simulink model "backlashcomptest"  (R2016a)
settings: Solver=VariableStepAuto  StartTime=0.0  StopTime=100  RelTol=1e-3
settings Model: Creator=julianleland  LastModifiedBy=julianleland

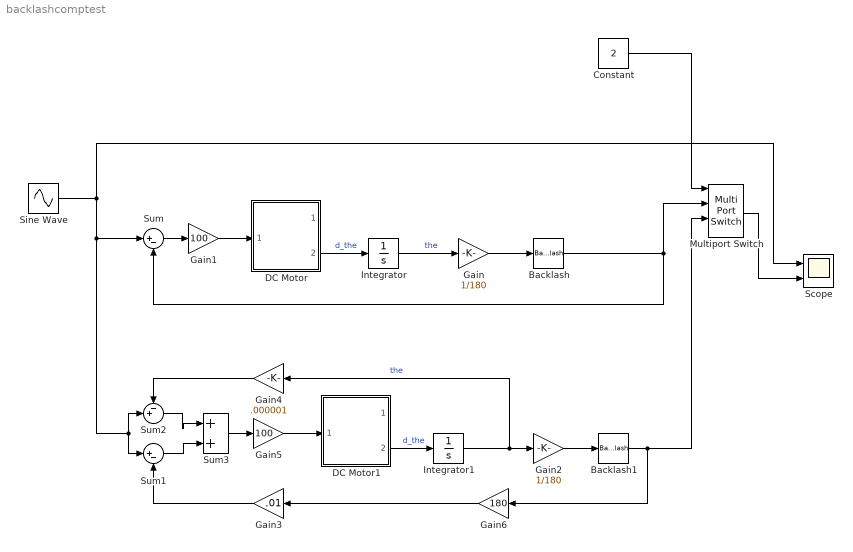
== system backlashcomptest ==
  Backlash : Backlash  BacklashWidth=10
  Backlash1 : Backlash  BacklashWidth=10
  Constant : Constant  Value=2
  DC Motor : Subsystem  mask(DC Motor){R=1, L=1, Q=2}
      mask prompts: R "Winding Resistance (ohms)"; L "Winding Inductance (mH)"; Q "Q Variable"
      mask help: From MIT Simulink Tutorial IAP 2017, Session 2. Provides basic model of DC motor using Kirchoff & Newton's laws.
      mask init:
      | J = R*L/Q
      | b = 1
      | k = 1
      | K = 1
      mask Help: See Julian with questions.
  DC Motor1 : Subsystem  mask(DC Motor){R=1, L=1, Q=2}
      mask prompts: R "Winding Resistance (ohms)"; L "Winding Inductance (mH)"; Q "Q Variable"
      mask help: From MIT Simulink Tutorial IAP 2017, Session 2. Provides basic model of DC motor using Kirchoff & Newton's laws.
      mask init:
      | J = R*L/Q
      | b = 1
      | k = 1
      | K = 1
      mask Help: See Julian with questions.
  Gain : Gain  Gain=1/180
  Gain1 : Gain  Gain=100
  Gain2 : Gain  Gain=1/180
  Gain3 : Gain  Gain=.01
  Gain4 : Gain  Gain=.000001
  Gain5 : Gain  Gain=100
  Gain6 : Gain  Gain=180
  Integrator : Integrator
  Integrator1 : Integrator
  Multiport Switch : MultiPortSwitch
  Scope : Scope  NumInputPorts=2
  Sine Wave : Sin  Amplitude=50  Frequency=0.1  SampleTime=0
  Sum : Sum  Inputs=|+-
  Sum1 : Sum  Inputs=|+-
  Sum2 : Sum  Inputs=-+|
  Sum3 : Sum
  wires:
  Integrator/1 -> Gain/1  "the"
  DC Motor/2(Speed) -> Integrator/1  "d_the"
  Gain/1 -> Backlash/1
  Backlash/1 -> Multiport Switch/2, Sum/2
  Sum/1 -> Gain1/1
  Gain1/1 -> DC Motor/1(Voltage)
  Multiport Switch/1 -> Scope/2
  Constant/1 -> Multiport Switch/1
  Integrator1/1 -> Gain4/1, Gain2/1  "the"
  DC Motor1/2(Speed) -> Integrator1/1  "d_the"
  Gain2/1 -> Backlash1/1
  Sine Wave/1 -> Sum1/1, Sum2/2, Sum/1, Scope/1
  Backlash1/1 -> Gain6/1, Multiport Switch/3
  Gain4/1 -> Sum2/1
  Gain5/1 -> DC Motor1/1(Voltage)
  Gain3/1 -> Sum1/2
  Sum3/1 -> Gain5/1
  Sum2/1 -> Sum3/1
  Sum1/1 -> Sum3/2
  Gain6/1 -> Gain3/1

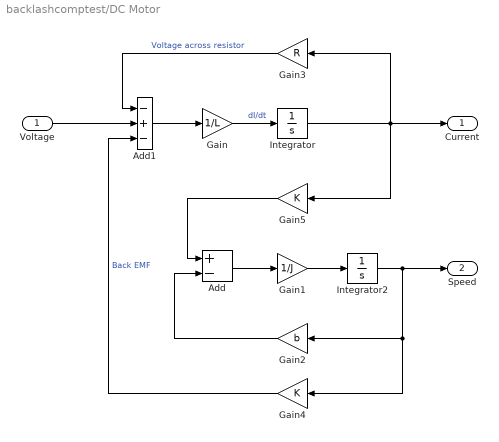
== system backlashcomptest/DC Motor ==
  Voltage : Inport
  Add : Sum  Inputs=+-
  Add1 : Sum  Inputs=-+-
  Gain : Gain  Gain=1/L
  Gain1 : Gain  Gain=1/J
  Gain2 : Gain  Gain=b
  Gain3 : Gain  Gain=R
  Gain4 : Gain  Gain=K
  Gain5 : Gain  Gain=K
  Integrator : Integrator
  Integrator2 : Integrator
  Current : Outport
  Speed : Outport  Port=2
  wires:
  Gain5/1 -> Add/1
  Voltage/1 -> Add1/2
  Gain1/1 -> Integrator2/1
  Integrator2/1 -> Speed/1, Gain4/1, Gain2/1
  Gain4/1 -> Add1/3  "Back EMF"
  Gain2/1 -> Add/2
  Add1/1 -> Gain/1
  Add/1 -> Gain1/1
  Gain3/1 -> Add1/1  "Voltage across resistor"
  Gain/1 -> Integrator/1  "dI/dt"
  Integrator/1 -> Current/1, Gain5/1, Gain3/1

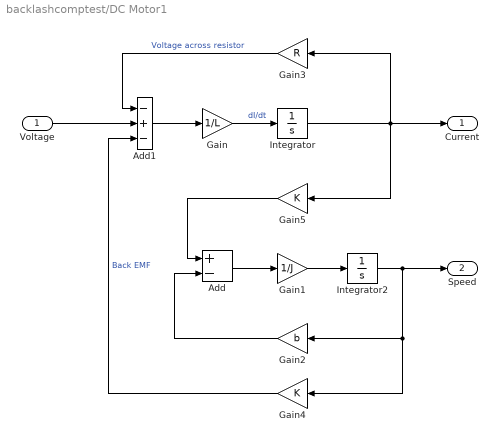
== system backlashcomptest/DC Motor1 ==
  Voltage : Inport
  Add : Sum  Inputs=+-
  Add1 : Sum  Inputs=-+-
  Gain : Gain  Gain=1/L
  Gain1 : Gain  Gain=1/J
  Gain2 : Gain  Gain=b
  Gain3 : Gain  Gain=R
  Gain4 : Gain  Gain=K
  Gain5 : Gain  Gain=K
  Integrator : Integrator
  Integrator2 : Integrator
  Current : Outport
  Speed : Outport  Port=2
  wires:
  Gain5/1 -> Add/1
  Voltage/1 -> Add1/2
  Gain1/1 -> Integrator2/1
  Integrator2/1 -> Speed/1, Gain4/1, Gain2/1
  Gain4/1 -> Add1/3  "Back EMF"
  Gain2/1 -> Add/2
  Add1/1 -> Gain/1
  Add/1 -> Gain1/1
  Gain3/1 -> Add1/1  "Voltage across resistor"
  Gain/1 -> Integrator/1  "dI/dt"
  Integrator/1 -> Current/1, Gain5/1, Gain3/1
